simulink model "hexsim"  (Simulink 8.6)
settings: Solver=ode45  StartTime=0.0  StopTime=100  FixedStep=0.002  RelTol=1e-3
InitFcn:
  | param
values from neighbouring files (symbols this model uses):
  colors = lines(length(row))    [adaptive_coefficients_figure.m]    (also in drawAircraft.m = [edgecolor; edgecolor; edgecolor; edgecolor; footprintcolor])
  V = V*R    [drawAircraft.m]
undefined symbols (not defined in the file or in its folder): attitude_controller, camera, compute_error, drawAircraft, F, forces_moments, geolocation, P, point_gimbal, position_controller
libraries: simulink x10, dspindex x1
settings Model: Creator=beard  LastModifiedBy=magiccjae
settings OptimizationCC: InitFltsAndDblsToZero=on
settings DebuggingCC: FcnCallInpInsideContextMsg=UseLocalSettings
settings ConfigComp: CovSFcnEnable=off

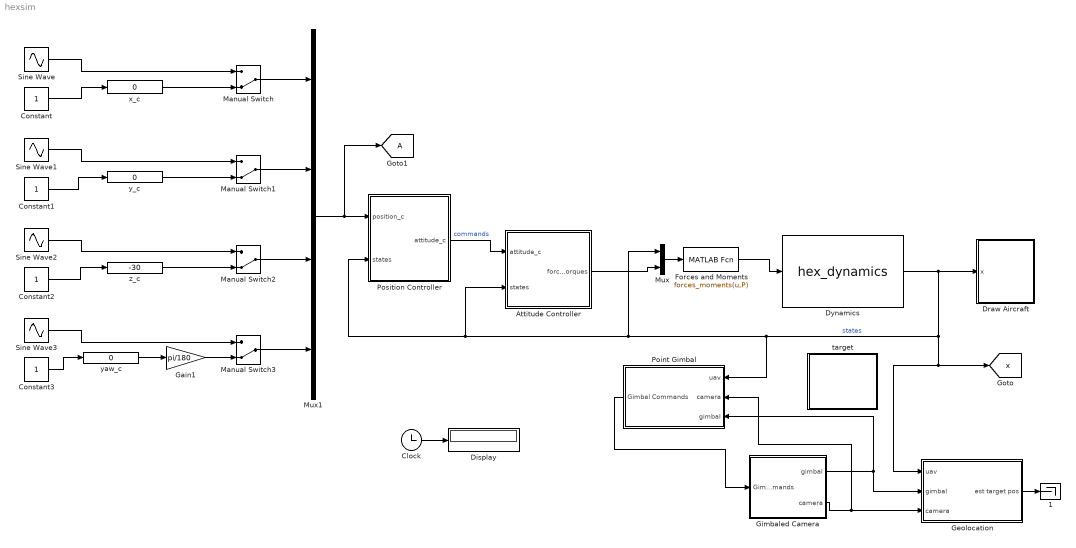
== system hexsim ==
  " 1" : Terminator
  Attitude Controller : Subsystem
      mask Display: image(imread('images/auto_pilot.jpg'))
  Clock : Clock
  Constant{,1..3} (4 alike) : Constant
  Display : Display
  Draw Aircraft : Subsystem
      mask Display: image(imread('images/tv.jpg'))
  Dynamics : S-Function  FunctionName=hex_dynamics  Parameters=P  SFunctionDeploymentMode=off  EnableBusSupport=off
      mask Display: image(imread('images/hexacopter.png'))
  Forces and Moments : MATLABFcn  MATLABFcn=forces_moments(u,P)  OutputDimensions=4*P.num_agents
  Gain1 : Gain  Gain=pi/180
  Geolocation : Subsystem
  Gimbaled Camera : Subsystem
      mask Display: image(imread('gimbal.jpg'))
  Manual Switch{,1..3} (4 alike) : ManualSwitch  CurrentSetting=0
  Mux : Mux  Inputs=2
  Mux1 : Mux
  Point Gimbal : Subsystem
  Position Controller : Subsystem
      mask Display: image(imread('images/ros.jpg'))
  Sine Wave : Sin  Amplitude=10  Frequency=0.5  Phase=pi/2  SampleTime=0
  Sine Wave1 : Sin  Amplitude=10  SampleTime=0
  Sine Wave2 : Sin  Amplitude=2  Frequency=0.5  SampleTime=0
  Sine Wave3 : Sin  Amplitude=180  Frequency=0.1  SampleTime=0
  target : Subsystem
      mask Display: image(imread('monstertruck.jpg'))
  x_c : simulink/Math Operations/Slider Gain  low=-1  gain=0  high=10
  y_c : simulink/Math Operations/Slider Gain  low=-30  gain=0  high=30
  yaw_c : simulink/Math Operations/Slider Gain  low=-180  gain=0  high=180
  z_c : simulink/Math Operations/Slider Gain  low=-90  gain=-30  high=0
  tag scope: A=global, x=global
  wires:
  Clock/1 -> Display/1
  Manual Switch/1 -> Mux1/1
  Manual Switch3/1 -> Mux1/4
  Manual Switch2/1 -> Mux1/3
  Manual Switch1/1 -> Mux1/2
  Sine Wave/1 -> Manual Switch/1
  Constant/1 -> x_c/1
  Sine Wave1/1 -> Manual Switch1/1
  Constant1/1 -> y_c/1
  Sine Wave2/1 -> Manual Switch2/1
  Constant2/1 -> z_c/1
  Sine Wave3/1 -> Manual Switch3/1
  Constant3/1 -> yaw_c/1
  Dynamics/1 -> Draw Aircraft/1(x), [x], Geolocation/1(uav), Point Gimbal/1(uav), Mux/1, Attitude Controller/2(states), Position Controller/2(states)  "states"
  Position Controller/1(attitude_c) -> Attitude Controller/1(attitude_c)  "commands"
  x_c/1 -> Manual Switch/2
  y_c/1 -> Manual Switch1/2
  z_c/1 -> Manual Switch2/2
  yaw_c/1 -> Gain1/1
  Gain1/1 -> Manual Switch3/2
  Forces and Moments/1 -> Dynamics/1
  Mux/1 -> Forces and Moments/1
  Attitude Controller/1(force_torques) -> Mux/2
  Gimbaled Camera/1(gimbal) -> Point Gimbal/3(gimbal), Geolocation/2(gimbal)
  Gimbaled Camera/2(camera) -> Point Gimbal/2(camera), Geolocation/3(camera)
  Geolocation/1(est target pos) -> " 1"/1
  Point Gimbal/1(Gimbal Commands) -> Gimbaled Camera/1(Gimbal Commands)
  Mux1/1 -> [A], Position Controller/1(position_c)

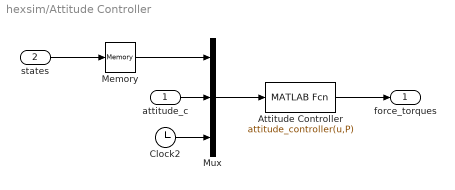
== system hexsim/Attitude Controller ==
  attitude_c : Inport
  states : Inport  Port=2
  Attitude Controller : MATLABFcn  MATLABFcn=attitude_controller(u,P)  OutputDimensions=4*P.num_agents  SampleTime=0.002
  Clock2 : Clock
  Memory : Memory
  Mux : Mux  Inputs=3
  force_torques : Outport
  wires:
  Clock2/1 -> Mux/3
  Mux/1 -> Attitude Controller/1
  Attitude Controller/1 -> force_torques/1
  states/1 -> Memory/1
  Memory/1 -> Mux/1
  attitude_c/1 -> Mux/2

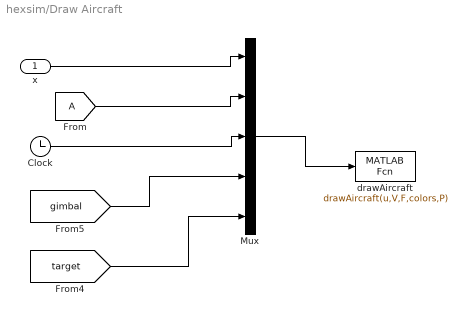
== system hexsim/Draw Aircraft ==
  x : Inport
  Clock : Clock
  Mux : Mux  Inputs=5
  drawAircraft : MATLABFcn  MATLABFcn=drawAircraft(u,V,F,colors,P)  OutputDimensions=0  SampleTime=0.1
  wires:
  x/1 -> Mux/1
  [A] -> Mux/2
  Mux/1 -> drawAircraft/1
  Clock/1 -> Mux/3
  [target] -> Mux/5
  [gimbal] -> Mux/4

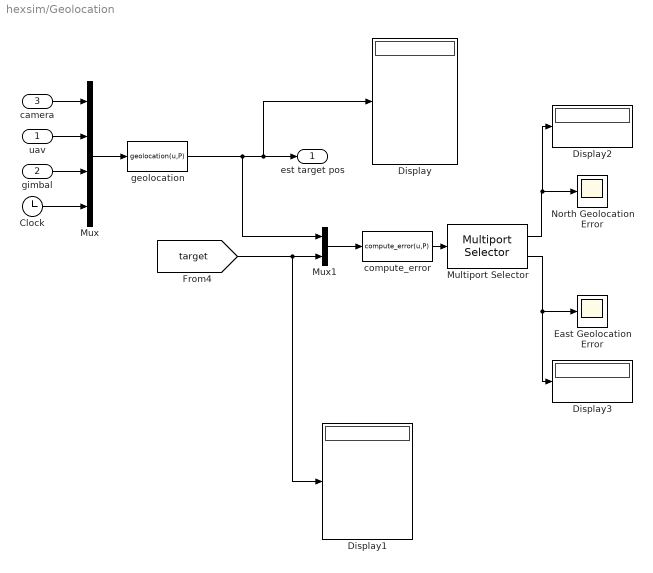
== system hexsim/Geolocation ==
  uav : Inport
  gimbal : Inport  Port=2
  camera : Inport  Port=3
  Clock : Clock
  Display{,1..3} (4 alike) : Display
  East Geolocation Error : Scope
  Multiport Selector : dspindex/Multiport Selector  rowsOrCols=Rows  idxCellArray={1:2:1+2*(P.num_agents-1),2:2:2+2*(P.num_agents-1)}  idxErrMode=Clip Index
  Mux : Mux
  Mux1 : Mux  Inputs=2
  North Geolocation Error : Scope
  "compute_error " : MATLABFcn  MATLABFcn=compute_error(u,P)  OutputDimensions=2*P.num_agents
  geolocation : MATLABFcn  MATLABFcn=geolocation(u,P)  OutputDimensions=3*P.num_agents  SampleTime=P.Ts
  est target pos : Outport
  wires:
  Clock/1 -> Mux/4
  Multiport Selector/1 -> Display2/1, North Geolocation Error/1
  [target] -> Display1/1, Mux1/2
  gimbal/1 -> Mux/3
  camera/1 -> Mux/1
  geolocation/1 -> Mux1/1, Display/1, est target pos/1
  uav/1 -> Mux/2
  Mux/1 -> geolocation/1
  Mux1/1 -> "compute_error "/1
  "compute_error "/1 -> Multiport Selector/1
  Multiport Selector/2 -> East Geolocation Error/1, Display3/1

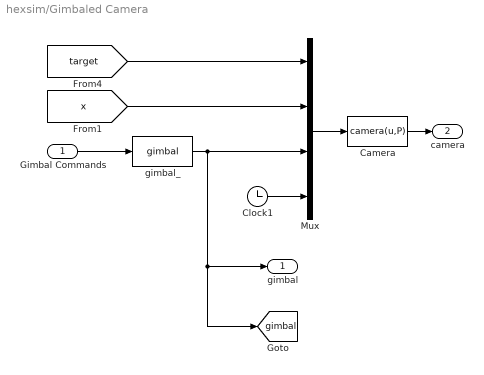
== system hexsim/Gimbaled Camera ==
  Gimbal Commands : Inport
  Camera : MATLABFcn  MATLABFcn=camera(u,P)  OutputDimensions=3*P.num_agents  SampleTime=1/P.cam_fps
  Clock1 : Clock
  Mux : Mux
  gimbal_ : S-Function  FunctionName=gimbal  Parameters=P  SFunctionDeploymentMode=off  EnableBusSupport=off
  gimbal : Outport
  camera : Outport  Port=2
  tag scope: gimbal=global
  wires:
  Mux/1 -> Camera/1
  [x] -> Mux/2
  Camera/1 -> camera/1
  [target] -> Mux/1
  Clock1/1 -> Mux/4
  Gimbal Commands/1 -> gimbal_/1
  gimbal_/1 -> Mux/3, gimbal/1, [gimbal]

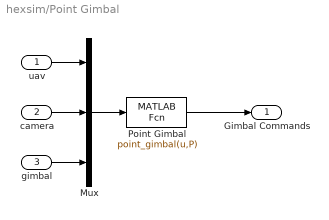
== system hexsim/Point Gimbal ==
  uav : Inport
  camera : Inport  Port=2
  gimbal : Inport  Port=3
  Mux : Mux  Inputs=3
  Point Gimbal : MATLABFcn  MATLABFcn=point_gimbal(u,P)  OutputDimensions=2*P.num_agents  SampleTime=P.Ts
  Gimbal Commands : Outport
  wires:
  Mux/1 -> Point Gimbal/1
  Point Gimbal/1 -> Gimbal Commands/1
  uav/1 -> Mux/1
  camera/1 -> Mux/2
  gimbal/1 -> Mux/3

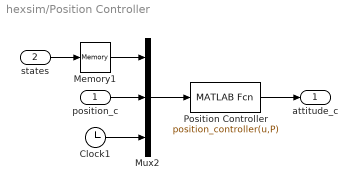
== system hexsim/Position Controller ==
  position_c : Inport
  states : Inport  Port=2
  Clock1 : Clock
  Memory1 : Memory
  Mux2 : Mux  Inputs=3
  Position Controller : MATLABFcn  MATLABFcn=position_controller(u,P)  OutputDimensions=4*P.num_agents  SampleTime=0.01
  attitude_c : Outport
  wires:
  Clock1/1 -> Mux2/3
  position_c/1 -> Mux2/2
  Position Controller/1 -> attitude_c/1
  Mux2/1 -> Position Controller/1
  states/1 -> Memory1/1
  Memory1/1 -> Mux2/1

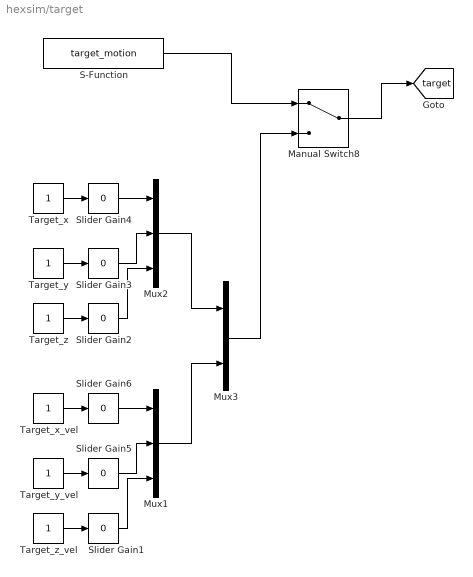
== system hexsim/target ==
  Manual Switch8 : ManualSwitch
  Mux1 : Mux  Inputs=3
  Mux2 : Mux  Inputs=3
  Mux3 : Mux  Inputs=2
  S-Function : S-Function  FunctionName=target_motion  Parameters=P  SFunctionDeploymentMode=off  EnableBusSupport=off
  Slider Gain{1..6} (6 alike) : simulink/Math Operations/Slider Gain  low=-180  gain=0  high=180
  "Target_x " : Constant
  Target_x_vel : Constant
  "Target_y " : Constant
  Target_y_vel : Constant
  Target_z : Constant
  Target_z_vel : Constant
  tag scope: target=global
  wires:
  Slider Gain4/1 -> Mux2/1
  "Target_x "/1 -> Slider Gain4/1
  "Target_y "/1 -> Slider Gain3/1
  Slider Gain3/1 -> Mux2/2
  Target_z/1 -> Slider Gain2/1
  Slider Gain2/1 -> Mux2/3
  Slider Gain6/1 -> Mux1/1
  Target_x_vel/1 -> Slider Gain6/1
  Target_y_vel/1 -> Slider Gain5/1
  Slider Gain5/1 -> Mux1/2
  Target_z_vel/1 -> Slider Gain1/1
  Slider Gain1/1 -> Mux1/3
  Mux2/1 -> Mux3/1
  Manual Switch8/1 -> [target]
  S-Function/1 -> Manual Switch8/1
  Mux3/1 -> Manual Switch8/2
  Mux1/1 -> Mux3/2
